simulink model "Iface"  (R2018b)
settings: Solver=FixedStepDiscrete  StartTime=0.0  StopTime=10.0  RelTol=1e-3
undefined symbols (not defined in the file or in its folder): boolSeqElement, intSeqElement, realSeqElement
settings Model: Creator=matlab  LastModifiedBy=matlab
settings DataIOCC: SaveOutput=off  SignalLogging=off  SaveTime=off
settings OptimizationCC: DefaultParameterBehavior=Inlined  EnhancedBackFolding=on  PassReuseOutputArgsAs=Individual arguments  OptimizeBlockOrder=speed  DifferentSizesBufferReuse=on  OptimizationCustomize=off
settings DebuggingCC: ParameterTunabilityLossMsg=error
settings SFSimCC: MATLABDynamicMemAlloc=off
settings RTWCC: SystemTargetFile=ert.tlc  TemplateMakefile=ert_default_tmf  PostCodeGenCommand=packNGo(buildInfo);  GenerateReport=on  IncludeHyperlinkInReport=on  LaunchReport=on  GenerateTraceInfo=on  GenerateTraceReport=on  GenerateTraceReportSl=on  GenerateTraceReportSf=on  GenerateTraceReportEml=on
settings CodeAppCC: ForceParamTrailComments=on  IgnoreCustomStorageClasses=off  OperatorAnnotations=on  SimulinkDataObjDesc=on  SFDataObjDesc=on  InsertBlockDesc=on
settings ERTTargetCC: TargetLangStandard=C99 (ISO)  GenerateSampleERTMain=on  InlinedParameterPlacement=NonHierarchical  ERTCustomFileTemplate=example_file_process.tlc

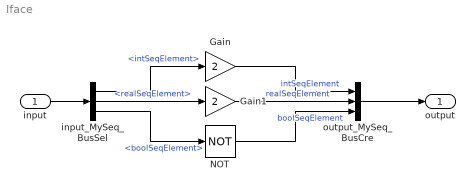
== system Iface ==
  input : Inport  OutDataTypeStr=Bus: MySeq  BusOutputAsStruct=on
  Gain : Gain  Gain=2  OutDataTypeStr=uint16
  Gain1 : Gain  Gain=2
  NOT : Logic  Operator=NOT  IconShape=distinctive  AllPortsSameDT=off  OutDataTypeStr=boolean
  input_MySeq_BusSel : BusSelector  OutputSignals=intSeqElement,realSeqElement,boolSeqElement
  output_MySeq_BusCre : BusCreator  Inputs=intSeqElement,realSeqElement,boolSeqElement  OutDataTypeStr=Bus: MySeq  NonVirtualBus=on
  output : Outport  OutDataTypeStr=Bus: MySeq  BusOutputAsStruct=on
  wires:
  input/1 -> input_MySeq_BusSel/1
  output_MySeq_BusCre/1 -> output/1
  input_MySeq_BusSel/1 -> Gain/1  "<intSeqElement>"
  input_MySeq_BusSel/2 -> Gain1/1  "<realSeqElement>"
  Gain1/1 -> output_MySeq_BusCre/2  "realSeqElement"
  Gain/1 -> output_MySeq_BusCre/1  "intSeqElement"
  input_MySeq_BusSel/3 -> NOT/1  "<boolSeqElement>"
  NOT/1 -> output_MySeq_BusCre/3  "boolSeqElement"
